simulink model "Washing_machine_Stateflow"  (R2024b)
settings: Solver=VariableStepAuto  StartTime=0.0  StopTime=inf  RelTol=1e-3
settings Model: Creator=kanith kumar  LastModifiedBy=kanith kumar

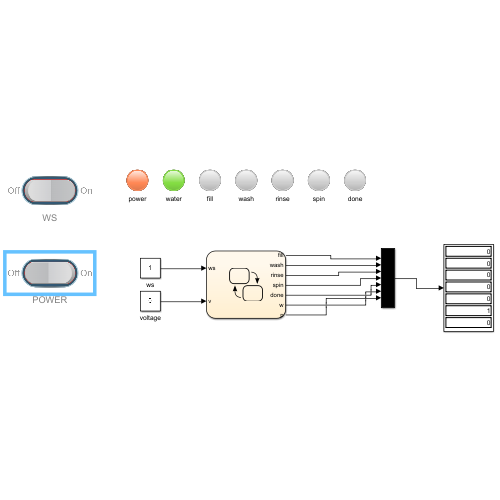
[thumbnail: Simulink's stored preview of the top-level diagram]
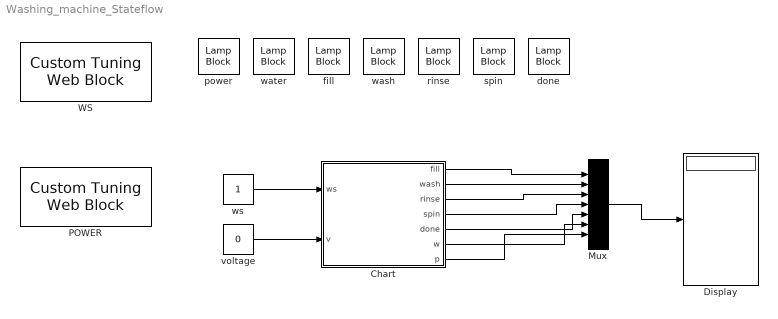
== system Washing_machine_Stateflow ==
  Chart : Stateflow chart  TreatAsAtomicUnit=on
  Display : Display
  Mux : Mux  Inputs=7
  POWER : CustomTuningWebBlock  LabelPosition=Hide  ShowInitialText=on  Configuration="{\"components\":[{\"name\":\"CustomSwitchStateComponent\",\"settings\":{\"position\":[0,0,1,1],\"states\":[{\"HitRegion\":{\"position\":[0,0,0.5,1]},\"Image\":{\"position\":[0.13,0,1,0.75],\"size\":[1,0.75],\"src\":\"data:image\\/svg+xml;base64,PHN2ZyB4bWxucz0iaHR0cDovL3d3dy53My5vcmcvMjAwMC9zdmciIHhtbG5zOnhsaW5rPSJodHRwOi8vd3d3LnczLm9yZy8xOTk5L3hsaW5rIiB2aWV3Qm94PSIwIDAgNzUgMjQuOCI+PGRlZnM+PHN0eWxlPi5jbHMtMXtmaWxsOnVybCgjcmFkaWFsLWdyYWRpZW50KTt9LmNscy0ye2ZpbGw6dXJsKCNyYWRpYWwtZ3JhZGllbnQtMik7fS5jbHMtM3tzdHJva2U6I2IyMDAwMDtzdHJva2Utd2lkdGg6MC4yNXB4O2ZpbGw6dXJsKCNsaW5lYXItZ3JhZGllbnQpO30uY2xzLTR7ZmlsbDp1cmwoI2xpbmVhci1ncmFkaWVudC0yKTt9LmNs ...(+3576 chars)\",\"srcOrientation\":\"Right\"},\"Label\":{\"color\":[0.5019607843137255,0.5019607843137255,0.5019607843137255],\"icon\":{\"size\":[0,0],\"src\":[],\"srcOrientation\":\"Right\"},\"iconOffset\":0,\"iconPlacement\":\"left\",\"opacity\":1,\"position\":[0.5,0.08],\"show\":true,\"text\":{\"content\":\"Off\",\"font\":\"Helvetica\"}},\"Value\":0},{\"HitRegion\":{\"position\":[0,0.5,0.5,1]},\"Image\":{\"position\":[0.13,0,1,0.75],\"size\":[1,0.75],\"src\":\"data:image\\/svg+xml;base64,PHN2ZyB4bWxucz0iaHR0cDovL3d3dy53My5vcmcvMjAwMC9zdmciIHhtbG5zOnhsaW5rPSJodHRwOi8vd3d3LnczLm9yZy8xOTk5L3hsaW5rIiB2aWV3Qm94PSIwIDAgNzUgMjQuOCI+PGRlZnM+PHN0eWxlPi5jbHMtMXtmaWxsOnVybCgjcmFkaWFsLWdyYWRpZW50KTt9LmNscy0ye2ZpbGw6dXJsKCNyYWRpYWwtZ3JhZGllbnQtMik7fS5jbHMtM3tzdHJva2U6I2IyMDAwMDtzdHJva2Utd2lkdGg6MC4yNXB4O2ZpbGw6dXJsKCNsaW5lYXItZ3JhZGllbnQpO30uY2xzLTR7ZmlsbDp1cmwoI2xpbmVhci1ncmFkaWVudC0yKTt9LmNs ...(+3520 chars)\",\"srcOrientation\":\"Right\"},\"Label\":{\"color\":[0.5019607843137255,0.5019607843137255,0.5019607843137255],\"icon\":{\"size\":[0,0],\"src\":[],\"srcOrientation\":\"Right\"},\"iconOffset\":0,\"iconPlacement\":\"left\",\"opacity\":1,\"position\":[0.5,0.92],\"show\":true,\"text\":{\"content\":\"On\",\"font\":\"Helvetica\"}},\"Value\":1}]}},{\"name\":\"BackgroundImageComponent\",\"settings\":{\"image\":{\"size\":[155,70],\"src\":\"default\",\"srcOrientation\":\"Right\"},\"position\":[0,0,1,1],\"scaleMode\":\"0\"}},{\"name\":\"ForegroundImageComponent\",\"settings\":{\"image\":{\"size\":[0,0],\"src\":\"default\",\"srcOrientation\":[]},\"isForeground\":1,\"position\":[0,0,1,1],\"scaleMode\":\"0\"}}],\"settings\":{\"BindingType\":\"param\",\"backgroundColor\":[0,0,255,\"1\"],\"backgroundOffset\":0.14,\"fixedAspectRatio\":\"on\",\"foregroundColor\":[234,234,234],\"showBackgroundColor\":false,\"variant\":\"rocker\",\"version\":\"R2024b\"},\"type\":\"Switch\"}"
  WS : CustomTuningWebBlock  LabelPosition=Hide  ShowInitialText=on  Configuration="{\"components\":[{\"name\":\"CustomSwitchStateComponent\",\"settings\":{\"position\":[0,0,1,1],\"states\":[{\"HitRegion\":{\"position\":[0,0,0.5,1]},\"Image\":{\"position\":[0.13,0,1,0.75],\"size\":[1,0.75],\"src\":\"data:image\\/svg+xml;base64,PHN2ZyB4bWxucz0iaHR0cDovL3d3dy53My5vcmcvMjAwMC9zdmciIHhtbG5zOnhsaW5rPSJodHRwOi8vd3d3LnczLm9yZy8xOTk5L3hsaW5rIiB2aWV3Qm94PSIwIDAgNzUgMjQuOCI+PGRlZnM+PHN0eWxlPi5jbHMtMXtmaWxsOnVybCgjcmFkaWFsLWdyYWRpZW50KTt9LmNscy0ye2ZpbGw6dXJsKCNyYWRpYWwtZ3JhZGllbnQtMik7fS5jbHMtM3tzdHJva2U6I2IyMDAwMDtzdHJva2Utd2lkdGg6MC4yNXB4O2ZpbGw6dXJsKCNsaW5lYXItZ3JhZGllbnQpO30uY2xzLTR7ZmlsbDp1cmwoI2xpbmVhci1ncmFkaWVudC0yKTt9LmNs ...(+3576 chars)\",\"srcOrientation\":\"Right\"},\"Label\":{\"color\":[0.5019607843137255,0.5019607843137255,0.5019607843137255],\"icon\":{\"size\":[0,0],\"src\":[],\"srcOrientation\":\"Right\"},\"iconOffset\":0,\"iconPlacement\":\"left\",\"opacity\":1,\"position\":[0.5,0.08],\"show\":true,\"text\":{\"content\":\"Off\",\"font\":\"Helvetica\"}},\"Value\":0},{\"HitRegion\":{\"position\":[0,0.5,0.5,1]},\"Image\":{\"position\":[0.13,0,1,0.75],\"size\":[1,0.75],\"src\":\"data:image\\/svg+xml;base64,PHN2ZyB4bWxucz0iaHR0cDovL3d3dy53My5vcmcvMjAwMC9zdmciIHhtbG5zOnhsaW5rPSJodHRwOi8vd3d3LnczLm9yZy8xOTk5L3hsaW5rIiB2aWV3Qm94PSIwIDAgNzUgMjQuOCI+PGRlZnM+PHN0eWxlPi5jbHMtMXtmaWxsOnVybCgjcmFkaWFsLWdyYWRpZW50KTt9LmNscy0ye2ZpbGw6dXJsKCNyYWRpYWwtZ3JhZGllbnQtMik7fS5jbHMtM3tzdHJva2U6I2IyMDAwMDtzdHJva2Utd2lkdGg6MC4yNXB4O2ZpbGw6dXJsKCNsaW5lYXItZ3JhZGllbnQpO30uY2xzLTR7ZmlsbDp1cmwoI2xpbmVhci1ncmFkaWVudC0yKTt9LmNs ...(+3520 chars)\",\"srcOrientation\":\"Right\"},\"Label\":{\"color\":[0.5019607843137255,0.5019607843137255,0.5019607843137255],\"icon\":{\"size\":[0,0],\"src\":[],\"srcOrientation\":\"Right\"},\"iconOffset\":0,\"iconPlacement\":\"left\",\"opacity\":1,\"position\":[0.5,0.92],\"show\":true,\"text\":{\"content\":\"On\",\"font\":\"Helvetica\"}},\"Value\":1}]}},{\"name\":\"BackgroundImageComponent\",\"settings\":{\"image\":{\"size\":[155,70],\"src\":\"default\",\"srcOrientation\":\"Right\"},\"position\":[0,0,1,1],\"scaleMode\":\"0\"}},{\"name\":\"ForegroundImageComponent\",\"settings\":{\"image\":{\"size\":[0,0],\"src\":\"default\",\"srcOrientation\":[]},\"isForeground\":1,\"position\":[0,0,1,1],\"scaleMode\":\"0\"}}],\"settings\":{\"BindingType\":\"param\",\"backgroundColor\":[0,0,255,\"1\"],\"backgroundOffset\":0.14,\"fixedAspectRatio\":\"on\",\"foregroundColor\":[234,234,234],\"showBackgroundColor\":false,\"variant\":\"rocker\",\"version\":\"R2024b\"},\"type\":\"Switch\"}"
  done : LampBlock  LabelPosition=Hide
  fill : LampBlock  LabelPosition=Hide
  power : LampBlock  LabelPosition=Hide
  rinse : LampBlock  LabelPosition=Hide
  spin : LampBlock  LabelPosition=Hide
  voltage : Constant  Value=0
  wash : LampBlock  LabelPosition=Hide
  water : LampBlock  LabelPosition=Hide
  ws : Constant
  wires:
  Chart/1(fill) -> Mux/1
  Chart/2(wash) -> Mux/2
  Chart/3(rinse) -> Mux/3
  Chart/4(spin) -> Mux/4
  Mux/1 -> Display/1
  Chart/5(done) -> Mux/5
  Chart/6(w) -> Mux/6
  Chart/7(p) -> Mux/7
  voltage/1 -> Chart/2(v)
  ws/1 -> Chart/1(ws)

== stateflow chart Washing_machine_Stateflow/Chart ==
  state Power_OFF1
    p=0;
    done=0;
  state Power_ON
    p=1;
  state Water_low
    w=0
  state Water_ch
  state Water_H
    w=1;
  state Done
    entry:
    spin=0;
    during:
    done=1;
  state Fill
    entry:
    during:
    fill=1;
  state Rinse
    entry:
    wash=0;
    during:
    rinse=1;
  state Wash
    entry:
    fill=0;
    during:
    wash=1;
  state Spin
    entry:
    rinse=0;
    during:
    spin=1;
  (default) -> Power_OFF1
  Power_OFF1 -> Power_ON : [v==1]
  Power_ON -> Power_OFF1 [order 1] : [v==0]
  Done -> Power_OFF1 : [after(10,sec)]
  Power_ON -> Water_ch [order 2]
  Water_low -> Power_OFF1
  Water_ch -> Water_H [order 1] : [ws==1]
  Water_ch -> Water_low [order 2] : [ws==0]
  Water_H -> Fill : [after(10,sec)]
  Spin -> Done : [after(10,sec)]
  Fill -> Wash : [after(10,sec)]
  Wash -> Rinse : [after(10,sec)]
  Rinse -> Spin : [after(10,sec)]
  data: fill output; wash output; rinse output; spin output; done output; ws input; v input; w output; p output
